simulink library "halin"  (R2021b)
settings: Solver=VariableStepAuto  StartTime=0.0  StopTime=10.0  RelTol=1e-3
undefined symbols (not defined in the file): KHAL_CAN1ABM1E2E_flg, KHAL_CAN1EPB1E2E_flg, KHAL_CAN1EPS1E2E_flg, KHAL_CAN1ESC1E2E_flg, KHAL_CAN1ESC5E2E_flg, KHAL_CAN3BMS1E2E_flg, KHAL_CAN3BMS6E2E_flg, KHAL_CAN3CCU1E2E_flg, KHAL_CAN3CCU2E2E_flg, KHAL_CAN3MCUNF1E2E_flg, KHAL_CAN3MCUNR1E2E_flg, KHAL_CAN3Shifter1E2E_flg, KHAL_CAN3Shifter2E2E_flg, KHAL_CAN6FCM2E2E_flg, KHAL_CAN6FCM4E2E_flg, TRUE
libraries: simulink x645, FVT_lib x212, hcu_lib x59
(part 7 of 23)

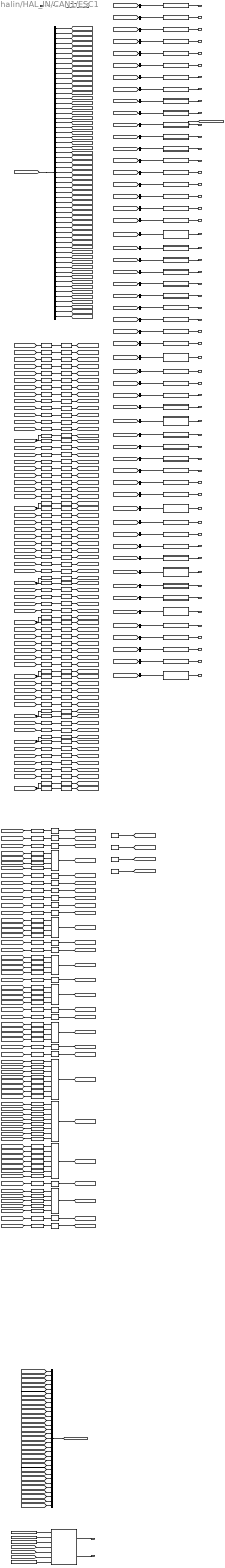
== system halin/HAL_IN/CAN1/ESC1 ==
  DT_CAN1_SG_ESC1 : Inport
  0x5F : Constant  Value=0x5F
  0xB3 : Constant  Value=0xB3
  ABSActive : Subsystem
  ABSFailed : Subsystem
  ABSWnlmpSta : Subsystem
  AVHActive : Subsystem
  AVHFailed : Subsystem
  AmberWnlmpSta : Subsystem
  BTCSActive : Subsystem
  BitwiseAND{,1..66} (67 alike) : simulink/Logic and Bit Operations/Bitwise Operator  logicop=AND  UseBitMask=on  BitMask=0xFF  BitMaskRealWorld=Stored Integer
  BitwiseOR{,1..2,4..9,11..12,14,16..17,19..20,24,26..27} (19 alike) : simulink/Logic and Bit Operations/Bitwise Operator  logicop=OR  UseBitMask=off  BitMask=bin2dec('11011001')  BitMaskRealWorld=Stored Integer
  BitwiseOR{3,10,13,15,18} (5 alike) : simulink/Logic and Bit Operations/Bitwise Operator  logicop=OR  UseBitMask=off  NumInputPorts=4  BitMask=bin2dec('11011001')  BitMaskRealWorld=Stored Integer
  BitwiseOR21 : simulink/Logic and Bit Operations/Bitwise Operator  logicop=OR  UseBitMask=off  NumInputPorts=8  BitMask=bin2dec('11011001')  BitMaskRealWorld=Stored Integer
  BitwiseOR22 : simulink/Logic and Bit Operations/Bitwise Operator  logicop=OR  UseBitMask=off  NumInputPorts=8  BitMask=bin2dec('11011001')  BitMaskRealWorld=Stored Integer
  BitwiseOR23 : simulink/Logic and Bit Operations/Bitwise Operator  logicop=OR  UseBitMask=off  NumInputPorts=7  BitMask=bin2dec('11011001')  BitMaskRealWorld=Stored Integer
  BitwiseOR25 : simulink/Logic and Bit Operations/Bitwise Operator  logicop=OR  UseBitMask=off  NumInputPorts=5  BitMask=bin2dec('11011001')  BitMaskRealWorld=Stored Integer
  DDM_CS&RC_Comparison : FVT_lib/hal/DDM_CS&RC_Comparison  MsgCycleTime=10
  Data Type Conversion{,1..66} (67 alike) : DataTypeConversion  OutDataTypeStr=uint8
  EBDActive : Subsystem
  EBDFailed : Subsystem
  ESC1CS : Subsystem
  ESC1RC : Subsystem
  ESCActive : Subsystem
  ESCBeepReq : Subsystem
  ESCFailed : Subsystem
  ESCOFFStatus : Subsystem
  ESCOfflmpSta : Subsystem
  ESCWnlmpSta : Subsystem
  ESSActive : Subsystem
  FrPTCSActive : Subsystem
  FrntAxlTrqReqDrv : Subsystem
  GRADE : Subsystem
  HBBActive : Subsystem
  HBBFailed : Subsystem
  HDDActive : Subsystem
  HDDFailed : Subsystem
  HSAActive : Subsystem
  HSAFailed : Subsystem
  KHAL_CAN1ESC1E2E_flg : Constant  Value=KHAL_CAN1ESC1E2E_flg
  LFPulseCount : Subsystem
  LFPulseCountV : Subsystem
  LFRawWhlSpeed : Subsystem
  LFRawWhlSpeedV : Subsystem
  LFWhlRotDir : Subsystem
  LRPulseCount : Subsystem
  LRPulseCountV : Subsystem
  LRRawWhlSpeed : Subsystem
  LRRawWhlSpeedV : Subsystem
  LRWhlRotDir : Subsystem
  LeftShift{,6,20,37,40,43} (6 alike) : ArithShift  BitShiftNumber=3  BitShiftDirection=Left
  LeftShift{1,16..17,33..34,36,47} (7 alike) : ArithShift  BitShiftNumber=7  BitShiftDirection=Left
  LeftShift{9..10,18,21,26,28,31..32,38,41..42,45,48,50} (14 alike) : ArithShift  BitShiftDirection=Left
  LeftShift{4,11,24,46} (4 alike) : ArithShift  BitShiftNumber=5  BitShiftDirection=Left
  LeftShift{2,8,12,22,25,44} (6 alike) : ArithShift  BitShiftNumber=6  BitShiftDirection=Left
  LeftShift{13,15,19,27,35,49} (6 alike) : ArithShift  BitShiftNumber=4  BitShiftDirection=Left
  LeftShift14 : ArithShift  BitShiftNumber=1  BitShiftDirection=Left
  LeftShift{5,7,23,29..30,39} (6 alike) : ArithShift  BitShiftNumber=2  BitShiftDirection=Left
  LeftShift3 : ArithShift  BitShiftNumber=1  BitShiftDirection=Left
  MessageRollingCounter : FVT_lib/hal/MessageRollingCounter  CounterMAX=14  task_time_ms=5  msg_time_ms=10
  Mux : Mux  Inputs=31
  PBAActive : Subsystem
  PBAFailed : Subsystem
  RFPulseCount : Subsystem
  RFPulseCountV : Subsystem
  RFRawWhlSpeed : Subsystem
  RFRawWhlSpeedV : Subsystem
  RFWhlRotDir : Subsystem
  RRPulseCount : Subsystem
  RRPulseCountV : Subsystem
  RRRawWhlSpeed : Subsystem
  RRRawWhlSpeedV : Subsystem
  RRWhlRotDir : Subsystem
  RearAxlTrqReqDrv : Subsystem
  RedWnlmpSta : Subsystem
  RightShift{,2,6,10,12} (5 alike) : ArithShift  BitShiftNumber=8
  RightShift{1,3,7,11,13} (5 alike) : ArithShift
  RightShift14 : ArithShift  BitShiftNumber=4
  RightShift15 : ArithShift  BitShiftNumber=-4
  RightShift4 : ArithShift  BitShiftNumber=4
  RightShift5 : ArithShift  BitShiftNumber=-4
  RightShift8 : ArithShift  BitShiftNumber=4
  RightShift9 : ArithShift  BitShiftNumber=-4
  RrPTCSActive : Subsystem
  TCSActive : Subsystem
  TCSFailed : Subsystem
  VehSpeed : Subsystem
  bus_selector : BusSelector  OutputSignals=CAN1_ABS_Active,CAN1_ABS_Failed,CAN1_ABS_WnlmpSta,CAN1_AVH_Active,CAN1_AVH_Failed,CAN1_Amber_WnlmpSta,CAN1_BTCS_Active,CAN1_EBD_Active,CAN1_EBD_Failed,CAN1_ESC1_CS,CAN1_ESC1_RC,CAN1_ESC_Active,CAN1_ESC_BeepReq,CAN1_ESC_EstVehSpd,CAN1_ESC_EstVehSpd_V,CAN1_ESC_Failed,CAN1_ESC_OFF_Status,CAN1_ESC_Off_lmpSta,CAN1_ESC_TSA_Active,CAN1_ESC_WnlmpSta,CAN1_ESS_Active,CAN1_Fr_PTCS_Active,CAN1_FrntAxlTrqReq_Drv,CAN1_GRADE,CAN1_HBB_Active,CAN1_HBB_Failed,CAN1_HDD_Active,CAN1_HDD_Failed,CAN1_HSA_Active,CAN1_HSA_Failed,CAN1_LF_PulseCount,CAN1_LF_PulseCount_V,CAN1_LF_RawWhlSpeed,CAN1_LF_RawWhlSpeed_V,CAN1_LF_WhlRotDir,CAN1_LR_PulseCount,CAN1_LR_PulseCount_V,CAN1_LR_RawWhlSpeed,CAN1_LR_RawWhlSpeed_V,CAN1_LR_WhlRotDir,CAN1_PBA_Active,CAN1_PBA_Failed,CAN1_RF_PulseCount,CAN1_RF_PulseCount_V,CAN1_RF_RawWhlSpeed,CAN1_RF_RawWhlSpeed_V,CAN1_RF_WhlRotDir,CAN1_RR_PulseCount,CAN1_RR_PulseCount_V,CAN1_RR_RawWhlSpeed,CAN1_RR_RawWhlSpeed_V,CAN1_RR_WhlRotDir,CAN1_RearAxlTrqReq_Drv,CAN1_Red_WnlmpSta,CAN1_Rr_PTCS_Active,CAN1_SystemVoltage,CAN1_TCS_Active,CAN1_TCS_Failed,CAN1_VehSpeed
  bus_selector1 : BusSelector  OutputSignals=CAN1_ABS_Active
  bus_selector10 : BusSelector  OutputSignals=CAN1_ESC1_CS
  bus_selector11 : BusSelector  OutputSignals=CAN1_ESC1_RC
  bus_selector12 : BusSelector  OutputSignals=CAN1_ESC_Active
  bus_selector13 : BusSelector  OutputSignals=CAN1_ESC_BeepReq
  bus_selector14 : BusSelector  OutputSignals=CAN1_ESC_Failed
  bus_selector15 : BusSelector  OutputSignals=CAN1_ESC_OFF_Status
  bus_selector16 : BusSelector  OutputSignals=CAN1_ESC_Off_lmpSta
  bus_selector17 : BusSelector  OutputSignals=CAN1_ESC_WnlmpSta
  bus_selector18 : BusSelector  OutputSignals=CAN1_ESS_Active
  bus_selector19 : BusSelector  OutputSignals=CAN1_Fr_PTCS_Active
  bus_selector2 : BusSelector  OutputSignals=CAN1_ABS_Failed
  bus_selector20 : BusSelector  OutputSignals=CAN1_FrntAxlTrqReq_Drv
  bus_selector21 : BusSelector  OutputSignals=CAN1_GRADE
  bus_selector22 : BusSelector  OutputSignals=CAN1_HBB_Active
  bus_selector23 : BusSelector  OutputSignals=CAN1_HBB_Failed
  bus_selector24 : BusSelector  OutputSignals=CAN1_HDD_Active
  bus_selector25 : BusSelector  OutputSignals=CAN1_HDD_Failed
  bus_selector26 : BusSelector  OutputSignals=CAN1_HSA_Active
  bus_selector27 : BusSelector  OutputSignals=CAN1_HSA_Failed
  bus_selector28 : BusSelector  OutputSignals=CAN1_LF_PulseCount
  bus_selector29 : BusSelector  OutputSignals=CAN1_LF_PulseCount_V
  bus_selector3 : BusSelector  OutputSignals=CAN1_ABS_WnlmpSta
  bus_selector30 : BusSelector  OutputSignals=CAN1_LF_RawWhlSpeed
  bus_selector31 : BusSelector  OutputSignals=CAN1_LF_RawWhlSpeed_V
  bus_selector32 : BusSelector  OutputSignals=CAN1_LF_WhlRotDir
  bus_selector33 : BusSelector  OutputSignals=CAN1_LR_PulseCount
  bus_selector34 : BusSelector  OutputSignals=CAN1_LR_PulseCount_V
  bus_selector35 : BusSelector  OutputSignals=CAN1_LR_RawWhlSpeed
  bus_selector36 : BusSelector  OutputSignals=CAN1_LR_RawWhlSpeed_V
  bus_selector37 : BusSelector  OutputSignals=CAN1_LR_WhlRotDir
  bus_selector38 : BusSelector  OutputSignals=CAN1_PBA_Active
  bus_selector39 : BusSelector  OutputSignals=CAN1_PBA_Failed
  bus_selector4 : BusSelector  OutputSignals=CAN1_AVH_Active
  bus_selector40 : BusSelector  OutputSignals=CAN1_RF_PulseCount
  bus_selector41 : BusSelector  OutputSignals=CAN1_RF_PulseCount_V
  bus_selector42 : BusSelector  OutputSignals=CAN1_RF_RawWhlSpeed
  bus_selector43 : BusSelector  OutputSignals=CAN1_RF_RawWhlSpeed_V
  bus_selector44 : BusSelector  OutputSignals=CAN1_RF_WhlRotDir
  bus_selector45 : BusSelector  OutputSignals=CAN1_RR_PulseCount
  bus_selector46 : BusSelector  OutputSignals=CAN1_RR_PulseCount_V
  bus_selector47 : BusSelector  OutputSignals=CAN1_RR_RawWhlSpeed
  bus_selector48 : BusSelector  OutputSignals=CAN1_RR_RawWhlSpeed_V
  bus_selector49 : BusSelector  OutputSignals=CAN1_RR_WhlRotDir
  bus_selector5 : BusSelector  OutputSignals=CAN1_AVH_Failed
  bus_selector50 : BusSelector  OutputSignals=CAN1_RearAxlTrqReq_Drv
  bus_selector51 : BusSelector  OutputSignals=CAN1_Red_WnlmpSta
  bus_selector52 : BusSelector  OutputSignals=CAN1_Rr_PTCS_Active
  bus_selector53 : BusSelector  OutputSignals=CAN1_TCS_Active
  bus_selector54 : BusSelector  OutputSignals=CAN1_TCS_Failed
  bus_selector55 : BusSelector  OutputSignals=CAN1_VehSpeed
  bus_selector6 : BusSelector  OutputSignals=CAN1_Amber_WnlmpSta
  bus_selector7 : BusSelector  OutputSignals=CAN1_BTCS_Active
  bus_selector8 : BusSelector  OutputSignals=CAN1_EBD_Active
  bus_selector9 : BusSelector  OutputSignals=CAN1_EBD_Failed
  constant{,1..3} (4 alike) : Constant  Value=0x0  OutDataTypeStr=uint8
  VHAL_ESC1CSErr_flg : Outport
  VHAL_ESC1RCErr_flg : Outport  Port=2
  VHAL_ABSActive_flg : Outport  Port=3
  VHAL_ABSFailed_flg : Outport  Port=4
  VHAL_ABSWnlmpSta_flg : Outport  Port=5
  VHAL_AVHActive_flg : Outport  Port=6
  VHAL_AVHFailed_flg : Outport  Port=7
  VHAL_AmberWnlmpSta_flg : Outport  Port=8
  VHAL_BTCSActive_flg : Outport  Port=9
  VHAL_EBDActive_flg : Outport  Port=10
  VHAL_EBDFailed_flg : Outport  Port=11
  VHAL_ESC1CS_enum : Outport  Port=12
  VHAL_ESC1RC_enum : Outport  Port=13
  VHAL_ESCActive_flg : Outport  Port=14
  VHAL_ESCBeepReq_flg : Outport  Port=15
  VHAL_ESCFailed_flg : Outport  Port=16
  VHAL_ESCOFFStatus_enum : Outport  Port=17
  VHAL_ESCOfflmpSta_flg : Outport  Port=18
  VHAL_ESCWnlmpSta_enum : Outport  Port=19
  VHAL_ESSActive_flg : Outport  Port=20
  VHAL_FrPTCSActive_flg : Outport  Port=21
  VHAL_FrntAxlTrqReqDrv_Nm : Outport  Port=22
  VHAL_GRADE_Deg : Outport  Port=23
  VHAL_HBBActive_flg : Outport  Port=24
  VHAL_HBBFailed_flg : Outport  Port=25
  VHAL_HDDActive_flg : Outport  Port=26
  VHAL_HDDFailed_flg : Outport  Port=27
  VHAL_HSAActive_flg : Outport  Port=28
  VHAL_HSAFailed_flg : Outport  Port=29
  VHAL_LFPulseCount_enum : Outport  Port=30
  VHAL_LFPulseCountV_flg : Outport  Port=31
  VHAL_LFRawWhlSpeed_kph : Outport  Port=32
  VHAL_LFRawWhlSpeedV_flg : Outport  Port=33
  VHAL_LFWhlRotDir_enum : Outport  Port=34
  VHAL_LRPulseCount_enum : Outport  Port=35
  VHAL_LRPulseCountV_flg : Outport  Port=36
  VHAL_LRRawWhlSpeed_kph : Outport  Port=37
  VHAL_LRRawWhlSpeedV_flg : Outport  Port=38
  VHAL_LRWhlRotDir_enum : Outport  Port=39
  VHAL_PBAActive_flg : Outport  Port=40
  VHAL_PBAFailed_flg : Outport  Port=41
  VHAL_RFPulseCount_enum : Outport  Port=42
  VHAL_RFPulseCountV_flg : Outport  Port=43
  VHAL_RFRawWhlSpeed_kph : Outport  Port=44
  VHAL_RFRawWhlSpeedV_flg : Outport  Port=45
  VHAL_RFWhlRotDir_enum : Outport  Port=46
  VHAL_RRPulseCount_enum : Outport  Port=47
  VHAL_RRPulseCountV_flg : Outport  Port=48
  VHAL_RRRawWhlSpeed_kph : Outport  Port=49
  VHAL_RRRawWhlSpeedV_flg : Outport  Port=50
  VHAL_RRWhlRotDir_enum : Outport  Port=51
  VHAL_RearAxlTrqReqDrv_Nm : Outport  Port=52
  VHAL_RedWnlmpSta_flg : Outport  Port=53
  VHAL_RrPTCSActive_flg : Outport  Port=54
  VHAL_TCSActive_flg : Outport  Port=55
  VHAL_TCSFailed_flg : Outport  Port=56
  VHAL_VehSpeed_kph : Outport  Port=57
  wires:
  DT_CAN1_SG_ESC1/1 -> [DT_CAN1_SG_ESC1]
  [DT_CAN1_SG_ESC1] -> bus_selector/1
  bus_selector/1 -> [CAN1_ABS_Active]  "<CAN1_ABS_Active>"
  [CAN1_ABS_Active] -> LeftShift/1
  LeftShift/1 -> BitwiseAND/1
  BitwiseAND/1 -> [Byte_23_CAN1_ABS_Active]
  bus_selector/2 -> [CAN1_ABS_Failed]  "<CAN1_ABS_Failed>"
  [CAN1_ABS_Failed] -> LeftShift1/1
  LeftShift1/1 -> BitwiseAND1/1
  BitwiseAND1/1 -> [Byte_22_CAN1_ABS_Failed]
  bus_selector/3 -> [CAN1_ABS_WnlmpSta]  "<CAN1_ABS_WnlmpSta>"
  [CAN1_ABS_WnlmpSta] -> LeftShift2/1
  LeftShift2/1 -> BitwiseAND2/1
  BitwiseAND2/1 -> [Byte_25_CAN1_ABS_WnlmpSta]
  bus_selector/4 -> [CAN1_AVH_Active]  "<CAN1_AVH_Active>"
  [CAN1_AVH_Active] -> LeftShift3/1
  LeftShift3/1 -> BitwiseAND3/1
  BitwiseAND3/1 -> [Byte_22_CAN1_AVH_Active]
  bus_selector/5 -> [CAN1_AVH_Failed]  "<CAN1_AVH_Failed>"
  [CAN1_AVH_Failed] -> LeftShift4/1
  LeftShift4/1 -> BitwiseAND4/1
  BitwiseAND4/1 -> [Byte_21_CAN1_AVH_Failed]
  bus_selector/6 -> [CAN1_Amber_WnlmpSta]  "<CAN1_Amber_WnlmpSta>"
  [CAN1_Amber_WnlmpSta] -> LeftShift5/1
  LeftShift5/1 -> BitwiseAND5/1
  BitwiseAND5/1 -> [Byte_22_CAN1_Amber_WnlmpSta]
  bus_selector/7 -> [CAN1_BTCS_Active]  "<CAN1_BTCS_Active>"
  [CAN1_BTCS_Active] -> LeftShift6/1
  LeftShift6/1 -> BitwiseAND6/1
  BitwiseAND6/1 -> [Byte_22_CAN1_BTCS_Active]
  bus_selector/8 -> [CAN1_EBD_Active]  "<CAN1_EBD_Active>"
  [CAN1_EBD_Active] -> LeftShift7/1
  LeftShift7/1 -> BitwiseAND7/1
  BitwiseAND7/1 -> [Byte_23_CAN1_EBD_Active]
  bus_selector/9 -> [CAN1_EBD_Failed]  "<CAN1_EBD_Failed>"
  [CAN1_EBD_Failed] -> LeftShift8/1
  LeftShift8/1 -> BitwiseAND8/1
  BitwiseAND8/1 -> [Byte_22_CAN1_EBD_Failed]
  bus_selector/10 -> [CAN1_ESC1_CS]  "<CAN1_ESC1_CS>"
  [CAN1_ESC1_CS] -> LeftShift9/1
  LeftShift9/1 -> BitwiseAND9/1
  BitwiseAND9/1 -> [Byte_0_CAN1_ESC1_CS]
  bus_selector/11 -> [CAN1_ESC1_RC]  "<CAN1_ESC1_RC>"
  [CAN1_ESC1_RC] -> LeftShift10/1
  LeftShift10/1 -> BitwiseAND10/1
  BitwiseAND10/1 -> [Byte_1_CAN1_ESC1_RC]
  bus_selector/12 -> [CAN1_ESC_Active]  "<CAN1_ESC_Active>"
  [CAN1_ESC_Active] -> LeftShift11/1
  LeftShift11/1 -> BitwiseAND11/1
  BitwiseAND11/1 -> [Byte_23_CAN1_ESC_Active]
  bus_selector/13 -> [CAN1_ESC_BeepReq]  "<CAN1_ESC_BeepReq>"
  [CAN1_ESC_BeepReq] -> LeftShift12/1
  LeftShift12/1 -> BitwiseAND12/1
  BitwiseAND12/1 -> [Byte_18_CAN1_ESC_BeepReq]
  bus_selector/14 -> [CAN1_ESC_EstVehSpd]  "<CAN1_ESC_EstVehSpd>"
  [CAN1_ESC_EstVehSpd] -> RightShift/1, RightShift1/1
  RightShift/1 -> BitwiseAND13/1
  BitwiseAND13/1 -> [Byte_25_CAN1_ESC_EstVehSpd]
  RightShift1/1 -> BitwiseAND14/1
  BitwiseAND14/1 -> [Byte_26_CAN1_ESC_EstVehSpd]
  bus_selector/15 -> [CAN1_ESC_EstVehSpd_V]  "<CAN1_ESC_EstVehSpd_V>"
  [CAN1_ESC_EstVehSpd_V] -> LeftShift13/1
  LeftShift13/1 -> BitwiseAND15/1
  BitwiseAND15/1 -> [Byte_25_CAN1_ESC_EstVehSpd_V]
  bus_selector/16 -> [CAN1_ESC_Failed]  "<CAN1_ESC_Failed>"
  [CAN1_ESC_Failed] -> LeftShift14/1
  LeftShift14/1 -> BitwiseAND16/1
  BitwiseAND16/1 -> [Byte_21_CAN1_ESC_Failed]
  bus_selector/17 -> [CAN1_ESC_OFF_Status]  "<CAN1_ESC_OFF_Status>"
  [CAN1_ESC_OFF_Status] -> LeftShift15/1
  LeftShift15/1 -> BitwiseAND17/1
  BitwiseAND17/1 -> [Byte_18_CAN1_ESC_OFF_Status]
  bus_selector/18 -> [CAN1_ESC_Off_lmpSta]  "<CAN1_ESC_Off_lmpSta>"
  [CAN1_ESC_Off_lmpSta] -> LeftShift16/1
  LeftShift16/1 -> BitwiseAND18/1
  BitwiseAND18/1 -> [Byte_25_CAN1_ESC_Off_lmpSta]
  bus_selector/19 -> [CAN1_ESC_TSA_Active]  "<CAN1_ESC_TSA_Active>"
  [CAN1_ESC_TSA_Active] -> LeftShift17/1
  LeftShift17/1 -> BitwiseAND19/1
  BitwiseAND19/1 -> [Byte_27_CAN1_ESC_TSA_Active]
  bus_selector/20 -> [CAN1_ESC_WnlmpSta]  "<CAN1_ESC_WnlmpSta>"
  [CAN1_ESC_WnlmpSta] -> LeftShift18/1
  LeftShift18/1 -> BitwiseAND20/1
  BitwiseAND20/1 -> [Byte_23_CAN1_ESC_WnlmpSta]
  bus_selector/21 -> [CAN1_ESS_Active]  "<CAN1_ESS_Active>"
  [CAN1_ESS_Active] -> LeftShift19/1
  LeftShift19/1 -> BitwiseAND21/1
  BitwiseAND21/1 -> [Byte_22_CAN1_ESS_Active]
  bus_selector/22 -> [CAN1_Fr_PTCS_Active]  "<CAN1_Fr_PTCS_Active>"
  [CAN1_Fr_PTCS_Active] -> LeftShift20/1
  LeftShift20/1 -> BitwiseAND22/1
  BitwiseAND22/1 -> [Byte_3_CAN1_Fr_PTCS_Active]
  bus_selector/23 -> [CAN1_FrntAxlTrqReq_Drv]  "<CAN1_FrntAxlTrqReq_Drv>"
  [CAN1_FrntAxlTrqReq_Drv] -> RightShift2/1, RightShift3/1
  RightShift2/1 -> BitwiseAND23/1
  BitwiseAND23/1 -> [Byte_4_CAN1_FrntAxlTrqReq_Drv]
  RightShift3/1 -> BitwiseAND24/1
  BitwiseAND24/1 -> [Byte_5_CAN1_FrntAxlTrqReq_Drv]
  bus_selector/24 -> [CAN1_GRADE]  "<CAN1_GRADE>"
  [CAN1_GRADE] -> LeftShift21/1
  LeftShift21/1 -> BitwiseAND25/1
  BitwiseAND25/1 -> [Byte_24_CAN1_GRADE]
  bus_selector/25 -> [CAN1_HBB_Active]  "<CAN1_HBB_Active>"
  [CAN1_HBB_Active] -> LeftShift22/1
  LeftShift22/1 -> BitwiseAND26/1
  BitwiseAND26/1 -> [Byte_23_CAN1_HBB_Active]
  bus_selector/26 -> [CAN1_HBB_Failed]  "<CAN1_HBB_Failed>"
  [CAN1_HBB_Failed] -> LeftShift23/1
  LeftShift23/1 -> BitwiseAND27/1
  BitwiseAND27/1 -> [Byte_21_CAN1_HBB_Failed]
  bus_selector/27 -> [CAN1_HDD_Active]  "<CAN1_HDD_Active>"
  [CAN1_HDD_Active] -> LeftShift24/1
  LeftShift24/1 -> BitwiseAND28/1
  BitwiseAND28/1 -> [Byte_22_CAN1_HDD_Active]
  bus_selector/28 -> [CAN1_HDD_Failed]  "<CAN1_HDD_Failed>"
  [CAN1_HDD_Failed] -> LeftShift25/1
  LeftShift25/1 -> BitwiseAND29/1
  BitwiseAND29/1 -> [Byte_21_CAN1_HDD_Failed]
  bus_selector/29 -> [CAN1_HSA_Active]  "<CAN1_HSA_Active>"
  [CAN1_HSA_Active] -> LeftShift26/1
  LeftShift26/1 -> BitwiseAND30/1
  BitwiseAND30/1 -> [Byte_22_CAN1_HSA_Active]
  bus_selector/30 -> [CAN1_HSA_Failed]  "<CAN1_HSA_Failed>"
  [CAN1_HSA_Failed] -> LeftShift27/1
  LeftShift27/1 -> BitwiseAND31/1
  BitwiseAND31/1 -> [Byte_21_CAN1_HSA_Failed]
  bus_selector/31 -> [CAN1_LF_PulseCount]  "<CAN1_LF_PulseCount>"
  [CAN1_LF_PulseCount] -> LeftShift28/1
  LeftShift28/1 -> BitwiseAND32/1
  BitwiseAND32/1 -> [Byte_11_CAN1_LF_PulseCount]
  bus_selector/32 -> [CAN1_LF_PulseCount_V]  "<CAN1_LF_PulseCount_V>"
  [CAN1_LF_PulseCount_V] -> LeftShift29/1
  LeftShift29/1 -> BitwiseAND33/1
  BitwiseAND33/1 -> [Byte_10_CAN1_LF_PulseCount_V]
  bus_selector/33 -> [CAN1_LF_RawWhlSpeed]  "<CAN1_LF_RawWhlSpeed>"
  [CAN1_LF_RawWhlSpeed] -> RightShift4/1, RightShift5/1
  RightShift4/1 -> BitwiseAND34/1
  BitwiseAND34/1 -> [Byte_12_CAN1_LF_RawWhlSpeed]
  RightShift5/1 -> BitwiseAND35/1
  BitwiseAND35/1 -> [Byte_13_CAN1_LF_RawWhlSpeed]
  bus_selector/34 -> [CAN1_LF_RawWhlSpeed_V]  "<CAN1_LF_RawWhlSpeed_V>"
  [CAN1_LF_RawWhlSpeed_V] -> LeftShift30/1
  LeftShift30/1 -> BitwiseAND36/1
  BitwiseAND36/1 -> [Byte_13_CAN1_LF_RawWhlSpeed_V]
  bus_selector/35 -> [CAN1_LF_WhlRotDir]  "<CAN1_LF_WhlRotDir>"
  [CAN1_LF_WhlRotDir] -> LeftShift31/1
  LeftShift31/1 -> BitwiseAND37/1
  BitwiseAND37/1 -> [Byte_10_CAN1_LF_WhlRotDir]
  bus_selector/36 -> [CAN1_LR_PulseCount]  "<CAN1_LR_PulseCount>"
  [CAN1_LR_PulseCount] -> LeftShift32/1
  LeftShift32/1 -> BitwiseAND38/1
  BitwiseAND38/1 -> [Byte_17_CAN1_LR_PulseCount]
  bus_selector/37 -> [CAN1_LR_PulseCount_V]  "<CAN1_LR_PulseCount_V>"
  [CAN1_LR_PulseCount_V] -> LeftShift33/1
  LeftShift33/1 -> BitwiseAND39/1
  BitwiseAND39/1 -> [Byte_15_CAN1_LR_PulseCount_V]
  bus_selector/38 -> [CAN1_LR_RawWhlSpeed]  "<CAN1_LR_RawWhlSpeed>"
  [CAN1_LR_RawWhlSpeed] -> RightShift6/1, RightShift7/1
  RightShift6/1 -> BitwiseAND40/1
  BitwiseAND40/1 -> [Byte_18_CAN1_LR_RawWhlSpeed]
  RightShift7/1 -> BitwiseAND41/1
  BitwiseAND41/1 -> [Byte_19_CAN1_LR_RawWhlSpeed]
  bus_selector/39 -> [CAN1_LR_RawWhlSpeed_V]  "<CAN1_LR_RawWhlSpeed_V>"
  [CAN1_LR_RawWhlSpeed_V] -> LeftShift34/1
  LeftShift34/1 -> BitwiseAND42/1
  BitwiseAND42/1 -> [Byte_18_CAN1_LR_RawWhlSpeed_V]
  bus_selector/40 -> [CAN1_LR_WhlRotDir]  "<CAN1_LR_WhlRotDir>"
  [CAN1_LR_WhlRotDir] -> LeftShift35/1
  LeftShift35/1 -> BitwiseAND43/1
  BitwiseAND43/1 -> [Byte_15_CAN1_LR_WhlRotDir]
  bus_selector/41 -> [CAN1_PBA_Active]  "<CAN1_PBA_Active>"
  [CAN1_PBA_Active] -> LeftShift36/1
  LeftShift36/1 -> BitwiseAND44/1
  BitwiseAND44/1 -> [Byte_23_CAN1_PBA_Active]
  bus_selector/42 -> [CAN1_PBA_Failed]  "<CAN1_PBA_Failed>"
  [CAN1_PBA_Failed] -> LeftShift37/1
  LeftShift37/1 -> BitwiseAND45/1
  BitwiseAND45/1 -> [Byte_21_CAN1_PBA_Failed]
  bus_selector/43 -> [CAN1_RF_PulseCount]  "<CAN1_RF_PulseCount>"
  [CAN1_RF_PulseCount] -> LeftShift38/1
  LeftShift38/1 -> BitwiseAND46/1
  BitwiseAND46/1 -> [Byte_8_CAN1_RF_PulseCount]
  bus_selector/44 -> [CAN1_RF_PulseCount_V]  "<CAN1_RF_PulseCount_V>"
  [CAN1_RF_PulseCount_V] -> LeftShift39/1
  LeftShift39/1 -> BitwiseAND47/1
  BitwiseAND47/1 -> [Byte_3_CAN1_RF_PulseCount_V]
  bus_selector/45 -> [CAN1_RF_RawWhlSpeed]  "<CAN1_RF_RawWhlSpeed>"
  [CAN1_RF_RawWhlSpeed] -> RightShift8/1, RightShift9/1
  RightShift8/1 -> BitwiseAND48/1
  BitwiseAND48/1 -> [Byte_9_CAN1_RF_RawWhlSpeed]
  RightShift9/1 -> BitwiseAND49/1
  BitwiseAND49/1 -> [Byte_10_CAN1_RF_RawWhlSpeed]
  bus_selector/46 -> [CAN1_RF_RawWhlSpeed_V]  "<CAN1_RF_RawWhlSpeed_V>"
  [CAN1_RF_RawWhlSpeed_V] -> LeftShift40/1
  LeftShift40/1 -> BitwiseAND50/1
  BitwiseAND50/1 -> [Byte_10_CAN1_RF_RawWhlSpeed_V]
  bus_selector/47 -> [CAN1_RF_WhlRotDir]  "<CAN1_RF_WhlRotDir>"
  [CAN1_RF_WhlRotDir] -> LeftShift41/1
  LeftShift41/1 -> BitwiseAND51/1
  BitwiseAND51/1 -> [Byte_3_CAN1_RF_WhlRotDir]
  bus_selector/48 -> [CAN1_RR_PulseCount]  "<CAN1_RR_PulseCount>"
  [CAN1_RR_PulseCount] -> LeftShift42/1
  LeftShift42/1 -> BitwiseAND52/1
  BitwiseAND52/1 -> [Byte_14_CAN1_RR_PulseCount]
  bus_selector/49 -> [CAN1_RR_PulseCount_V]  "<CAN1_RR_PulseCount_V>"
  [CAN1_RR_PulseCount_V] -> LeftShift43/1
  LeftShift43/1 -> BitwiseAND53/1
  BitwiseAND53/1 -> [Byte_13_CAN1_RR_PulseCount_V]
  bus_selector/50 -> [CAN1_RR_RawWhlSpeed]  "<CAN1_RR_RawWhlSpeed>"
  [CAN1_RR_RawWhlSpeed] -> RightShift10/1, RightShift11/1
  RightShift10/1 -> BitwiseAND54/1
  BitwiseAND54/1 -> [Byte_15_CAN1_RR_RawWhlSpeed]
  RightShift11/1 -> BitwiseAND55/1
  BitwiseAND55/1 -> [Byte_16_CAN1_RR_RawWhlSpeed]
  bus_selector/51 -> [CAN1_RR_RawWhlSpeed_V]  "<CAN1_RR_RawWhlSpeed_V>"
  [CAN1_RR_RawWhlSpeed_V] -> LeftShift44/1
  LeftShift44/1 -> BitwiseAND56/1
  BitwiseAND56/1 -> [Byte_15_CAN1_RR_RawWhlSpeed_V]
  bus_selector/52 -> [CAN1_RR_WhlRotDir]  "<CAN1_RR_WhlRotDir>"
  [CAN1_RR_WhlRotDir] -> LeftShift45/1
  LeftShift45/1 -> BitwiseAND57/1
  BitwiseAND57/1 -> [Byte_13_CAN1_RR_WhlRotDir]
  bus_selector/53 -> [CAN1_RearAxlTrqReq_Drv]  "<CAN1_RearAxlTrqReq_Drv>"
  [CAN1_RearAxlTrqReq_Drv] -> RightShift12/1, RightShift13/1
  RightShift12/1 -> BitwiseAND58/1
  BitwiseAND58/1 -> [Byte_6_CAN1_RearAxlTrqReq_Drv]
  RightShift13/1 -> BitwiseAND59/1
  BitwiseAND59/1 -> [Byte_7_CAN1_RearAxlTrqReq_Drv]
  bus_selector/54 -> [CAN1_Red_WnlmpSta]  "<CAN1_Red_WnlmpSta>"
  [CAN1_Red_WnlmpSta] -> LeftShift46/1
  LeftShift46/1 -> BitwiseAND60/1
  BitwiseAND60/1 -> [Byte_25_CAN1_Red_WnlmpSta]
  bus_selector/55 -> [CAN1_Rr_PTCS_Active]  "<CAN1_Rr_PTCS_Active>"
  [CAN1_Rr_PTCS_Active] -> LeftShift47/1
  LeftShift47/1 -> BitwiseAND61/1
  BitwiseAND61/1 -> [Byte_21_CAN1_Rr_PTCS_Active]
  bus_selector/56 -> [CAN1_SystemVoltage]  "<CAN1_SystemVoltage>"
  [CAN1_SystemVoltage] -> LeftShift48/1
  LeftShift48/1 -> BitwiseAND62/1
  BitwiseAND62/1 -> [Byte_20_CAN1_SystemVoltage]
  bus_selector/57 -> [CAN1_TCS_Active]  "<CAN1_TCS_Active>"
  [CAN1_TCS_Active] -> LeftShift49/1
  LeftShift49/1 -> BitwiseAND63/1
  BitwiseAND63/1 -> [Byte_23_CAN1_TCS_Active]
  bus_selector/58 -> [CAN1_TCS_Failed]  "<CAN1_TCS_Failed>"
  [CAN1_TCS_Failed] -> LeftShift50/1
  LeftShift50/1 -> BitwiseAND64/1
  BitwiseAND64/1 -> [Byte_21_CAN1_TCS_Failed]
  bus_selector/59 -> [CAN1_VehSpeed]  "<CAN1_VehSpeed>"
  [CAN1_VehSpeed] -> RightShift14/1, RightShift15/1
  RightShift14/1 -> BitwiseAND65/1
  BitwiseAND65/1 -> [Byte_2_CAN1_VehSpeed]
  RightShift15/1 -> BitwiseAND66/1
  BitwiseAND66/1 -> [Byte_3_CAN1_VehSpeed]
  Data Type Conversion/1 -> BitwiseOR/1
  [Byte_0_CAN1_ESC1_CS] -> Data Type Conversion/1
  BitwiseOR/1 -> [Byte_0]
  Data Type Conversion1/1 -> BitwiseOR1/1
  [Byte_1_CAN1_ESC1_RC] -> Data Type Conversion1/1
  BitwiseOR1/1 -> [Byte_1]
  Data Type Conversion2/1 -> BitwiseOR2/1
  [Byte_2_CAN1_VehSpeed] -> Data Type Conversion2/1
  BitwiseOR2/1 -> [Byte_2]
  Data Type Conversion3/1 -> BitwiseOR3/1
  [Byte_3_CAN1_Fr_PTCS_Active] -> Data Type Conversion3/1
  Data Type Conversion4/1 -> BitwiseOR3/2
  [Byte_3_CAN1_RF_PulseCount_V] -> Data Type Conversion4/1
  Data Type Conversion5/1 -> BitwiseOR3/3
  [Byte_3_CAN1_RF_WhlRotDir] -> Data Type Conversion5/1
  Data Type Conversion6/1 -> BitwiseOR3/4
  [Byte_3_CAN1_VehSpeed] -> Data Type Conversion6/1
  BitwiseOR3/1 -> [Byte_3]
  Data Type Conversion7/1 -> BitwiseOR4/1
  [Byte_4_CAN1_FrntAxlTrqReq_Drv] -> Data Type Conversion7/1
  BitwiseOR4/1 -> [Byte_4]
  Data Type Conversion8/1 -> BitwiseOR5/1
  [Byte_5_CAN1_FrntAxlTrqReq_Drv] -> Data Type Conversion8/1
  BitwiseOR5/1 -> [Byte_5]
  Data Type Conversion9/1 -> BitwiseOR6/1
  [Byte_6_CAN1_RearAxlTrqReq_Drv] -> Data Type Conversion9/1
  BitwiseOR6/1 -> [Byte_6]
  Data Type Conversion10/1 -> BitwiseOR7/1
  [Byte_7_CAN1_RearAxlTrqReq_Drv] -> Data Type Conversion10/1
  BitwiseOR7/1 -> [Byte_7]
  Data Type Conversion11/1 -> BitwiseOR8/1
  [Byte_8_CAN1_RF_PulseCount] -> Data Type Conversion11/1
  BitwiseOR8/1 -> [Byte_8]
  Data Type Conversion12/1 -> BitwiseOR9/1
  [Byte_9_CAN1_RF_RawWhlSpeed] -> Data Type Conversion12/1
  BitwiseOR9/1 -> [Byte_9]
  Data Type Conversion13/1 -> BitwiseOR10/1
  [Byte_10_CAN1_LF_PulseCount_V] -> Data Type Conversion13/1
  Data Type Conversion14/1 -> BitwiseOR10/2
  [Byte_10_CAN1_LF_WhlRotDir] -> Data Type Conversion14/1
  Data Type Conversion15/1 -> BitwiseOR10/3
  [Byte_10_CAN1_RF_RawWhlSpeed] -> Data Type Conversion15/1
  Data Type Conversion16/1 -> BitwiseOR10/4
  [Byte_10_CAN1_RF_RawWhlSpeed_V] -> Data Type Conversion16/1
  BitwiseOR10/1 -> [Byte_10]
  Data Type Conversion17/1 -> BitwiseOR11/1
  [Byte_11_CAN1_LF_PulseCount] -> Data Type Conversion17/1
  BitwiseOR11/1 -> [Byte_11]
  Data Type Conversion18/1 -> BitwiseOR12/1
  [Byte_12_CAN1_LF_RawWhlSpeed] -> Data Type Conversion18/1
  BitwiseOR12/1 -> [Byte_12]
  Data Type Conversion19/1 -> BitwiseOR13/1
  [Byte_13_CAN1_LF_RawWhlSpeed] -> Data Type Conversion19/1
  Data Type Conversion20/1 -> BitwiseOR13/2
  [Byte_13_CAN1_LF_RawWhlSpeed_V] -> Data Type Conversion20/1
  Data Type Conversion21/1 -> BitwiseOR13/3
  [Byte_13_CAN1_RR_PulseCount_V] -> Data Type Conversion21/1
  Data Type Conversion22/1 -> BitwiseOR13/4
  [Byte_13_CAN1_RR_WhlRotDir] -> Data Type Conversion22/1
  BitwiseOR13/1 -> [Byte_13]
  Data Type Conversion23/1 -> BitwiseOR14/1
  [Byte_14_CAN1_RR_PulseCount] -> Data Type Conversion23/1
  BitwiseOR14/1 -> [Byte_14]
  Data Type Conversion24/1 -> BitwiseOR15/1
  [Byte_15_CAN1_LR_PulseCount_V] -> Data Type Conversion24/1
  Data Type Conversion25/1 -> BitwiseOR15/2
  [Byte_15_CAN1_LR_WhlRotDir] -> Data Type Conversion25/1
  Data Type Conversion26/1 -> BitwiseOR15/3
  [Byte_15_CAN1_RR_RawWhlSpeed] -> Data Type Conversion26/1
  Data Type Conversion27/1 -> BitwiseOR15/4
  [Byte_15_CAN1_RR_RawWhlSpeed_V] -> Data Type Conversion27/1
  BitwiseOR15/1 -> [Byte_15]
  Data Type Conversion28/1 -> BitwiseOR16/1
  [Byte_16_CAN1_RR_RawWhlSpeed] -> Data Type Conversion28/1
  BitwiseOR16/1 -> [Byte_16]
  Data Type Conversion29/1 -> BitwiseOR17/1
  [Byte_17_CAN1_LR_PulseCount] -> Data Type Conversion29/1
  BitwiseOR17/1 -> [Byte_17]
  Data Type Conversion30/1 -> BitwiseOR18/1
  [Byte_18_CAN1_ESC_BeepReq] -> Data Type Conversion30/1
  Data Type Conversion31/1 -> BitwiseOR18/2
  [Byte_18_CAN1_ESC_OFF_Status] -> Data Type Conversion31/1
  Data Type Conversion32/1 -> BitwiseOR18/3
  [Byte_18_CAN1_LR_RawWhlSpeed] -> Data Type Conversion32/1
  Data Type Conversion33/1 -> BitwiseOR18/4
  [Byte_18_CAN1_LR_RawWhlSpeed_V] -> Data Type Conversion33/1
  BitwiseOR18/1 -> [Byte_18]
  Data Type Conversion34/1 -> BitwiseOR19/1
  [Byte_19_CAN1_LR_RawWhlSpeed] -> Data Type Conversion34/1
  BitwiseOR19/1 -> [Byte_19]
  Data Type Conversion35/1 -> BitwiseOR20/1
  [Byte_20_CAN1_SystemVoltage] -> Data Type Conversion35/1
  BitwiseOR20/1 -> [Byte_20]
  Data Type Conversion36/1 -> BitwiseOR21/1
  [Byte_21_CAN1_AVH_Failed] -> Data Type Conversion36/1
  Data Type Conversion37/1 -> BitwiseOR21/2
  [Byte_21_CAN1_ESC_Failed] -> Data Type Conversion37/1
  Data Type Conversion38/1 -> BitwiseOR21/3
  [Byte_21_CAN1_HBB_Failed] -> Data Type Conversion38/1
  Data Type Conversion39/1 -> BitwiseOR21/4
  [Byte_21_CAN1_HDD_Failed] -> Data Type Conversion39/1
  Data Type Conversion40/1 -> BitwiseOR21/5
  [Byte_21_CAN1_HSA_Failed] -> Data Type Conversion40/1
  Data Type Conversion41/1 -> BitwiseOR21/6
  [Byte_21_CAN1_PBA_Failed] -> Data Type Conversion41/1
  Data Type Conversion42/1 -> BitwiseOR21/7
  [Byte_21_CAN1_Rr_PTCS_Active] -> Data Type Conversion42/1
  Data Type Conversion43/1 -> BitwiseOR21/8
  [Byte_21_CAN1_TCS_Failed] -> Data Type Conversion43/1
  BitwiseOR21/1 -> [Byte_21]
  Data Type Conversion44/1 -> BitwiseOR22/1
  [Byte_22_CAN1_ABS_Failed] -> Data Type Conversion44/1
  Data Type Conversion45/1 -> BitwiseOR22/2
  [Byte_22_CAN1_AVH_Active] -> Data Type Conversion45/1
  Data Type Conversion46/1 -> BitwiseOR22/3
  [Byte_22_CAN1_Amber_WnlmpSta] -> Data Type Conversion46/1
  Data Type Conversion47/1 -> BitwiseOR22/4
  [Byte_22_CAN1_BTCS_Active] -> Data Type Conversion47/1
  Data Type Conversion48/1 -> BitwiseOR22/5
  [Byte_22_CAN1_EBD_Failed] -> Data Type Conversion48/1
  Data Type Conversion49/1 -> BitwiseOR22/6
  [Byte_22_CAN1_ESS_Active] -> Data Type Conversion49/1
  Data Type Conversion50/1 -> BitwiseOR22/7
  [Byte_22_CAN1_HDD_Active] -> Data Type Conversion50/1
  Data Type Conversion51/1 -> BitwiseOR22/8
  [Byte_22_CAN1_HSA_Active] -> Data Type Conversion51/1
  BitwiseOR22/1 -> [Byte_22]
  Data Type Conversion52/1 -> BitwiseOR23/1
  [Byte_23_CAN1_ABS_Active] -> Data Type Conversion52/1
  Data Type Conversion53/1 -> BitwiseOR23/2
  [Byte_23_CAN1_EBD_Active] -> Data Type Conversion53/1
  Data Type Conversion54/1 -> BitwiseOR23/3
  [Byte_23_CAN1_ESC_Active] -> Data Type Conversion54/1
  Data Type Conversion55/1 -> BitwiseOR23/4
  [Byte_23_CAN1_ESC_WnlmpSta] -> Data Type Conversion55/1
  Data Type Conversion56/1 -> BitwiseOR23/5
  [Byte_23_CAN1_HBB_Active] -> Data Type Conversion56/1
  Data Type Conversion57/1 -> BitwiseOR23/6
  [Byte_23_CAN1_PBA_Active] -> Data Type Conversion57/1
  Data Type Conversion58/1 -> BitwiseOR23/7
  [Byte_23_CAN1_TCS_Active] -> Data Type Conversion58/1
  BitwiseOR23/1 -> [Byte_23]
  Data Type Conversion59/1 -> BitwiseOR24/1
  [Byte_24_CAN1_GRADE] -> Data Type Conversion59/1
  BitwiseOR24/1 -> [Byte_24]
  Data Type Conversion60/1 -> BitwiseOR25/1
  [Byte_25_CAN1_ABS_WnlmpSta] -> Data Type Conversion60/1
  Data Type Conversion61/1 -> BitwiseOR25/2
  [Byte_25_CAN1_ESC_EstVehSpd] -> Data Type Conversion61/1
  Data Type Conversion62/1 -> BitwiseOR25/3
  [Byte_25_CAN1_ESC_EstVehSpd_V] -> Data Type Conversion62/1
  Data Type Conversion63/1 -> BitwiseOR25/4
  [Byte_25_CAN1_ESC_Off_lmpSta] -> Data Type Conversion63/1
  Data Type Conversion64/1 -> BitwiseOR25/5
  [Byte_25_CAN1_Red_WnlmpSta] -> Data Type Conversion64/1
  BitwiseOR25/1 -> [Byte_25]
  Data Type Conversion65/1 -> BitwiseOR26/1
  [Byte_26_CAN1_ESC_EstVehSpd] -> Data Type Conversion65/1
  BitwiseOR26/1 -> [Byte_26]
  Data Type Conversion66/1 -> BitwiseOR27/1
  [Byte_27_CAN1_ESC_TSA_Active] -> Data Type Conversion66/1
  BitwiseOR27/1 -> [Byte_27]
  constant/1 -> [Byte_28]
  constant1/1 -> [Byte_29]
  constant2/1 -> [Byte_30]
  constant3/1 -> [Byte_31]
  [Byte_1] -> Mux/1
  [Byte_2] -> Mux/2
  [Byte_3] -> Mux/3
  [Byte_4] -> Mux/4
  [Byte_5] -> Mux/5
  [Byte_6] -> Mux/6
  [Byte_7] -> Mux/7
  [Byte_8] -> Mux/8
  [Byte_9] -> Mux/9
  [Byte_10] -> Mux/10
  [Byte_11] -> Mux/11
  [Byte_12] -> Mux/12
  [Byte_13] -> Mux/13
  [Byte_14] -> Mux/14
  [Byte_15] -> Mux/15
  [Byte_16] -> Mux/16
  [Byte_17] -> Mux/17
  [Byte_18] -> Mux/18
  [Byte_19] -> Mux/19
  [Byte_20] -> Mux/20
  [Byte_21] -> Mux/21
  [Byte_22] -> Mux/22
  [Byte_23] -> Mux/23
  [Byte_24] -> Mux/24
  [Byte_25] -> Mux/25
  [Byte_26] -> Mux/26
  [Byte_27] -> Mux/27
  [Byte_28] -> Mux/28
  [Byte_29] -> Mux/29
  [Byte_30] -> Mux/30
  [Byte_31] -> Mux/31
  Mux/1 -> [VHAL_CAN1ESC1noCS_raw]
  KHAL_CAN1ESC1E2E_flg/1 -> DDM_CS&RC_Comparison/1
  0xB3/1 -> DDM_CS&RC_Comparison/2
  0x5F/1 -> DDM_CS&RC_Comparison/3
  [VHAL_CAN1ESC1noCS_raw] -> DDM_CS&RC_Comparison/4
  [Byte_0] -> DDM_CS&RC_Comparison/5
  [RC_ECU] -> DDM_CS&RC_Comparison/6
  MessageRollingCounter/1 -> DDM_CS&RC_Comparison/7
  DDM_CS&RC_Comparison/1 -> VHAL_ESC1CSErr_flg/1
  DDM_CS&RC_Comparison/2 -> VHAL_ESC1RCErr_flg/1
  [DT_CAN1_SG_ESC1] -> bus_selector1/1
  bus_selector1/1 -> ABSActive/1(ABS_Active)  "<CAN1_ABS_Active>"
  ABSActive/1(VHAL_ABSActive_flg) -> VHAL_ABSActive_flg/1
  [DT_CAN1_SG_ESC1] -> bus_selector2/1
  bus_selector2/1 -> ABSFailed/1(ABS_Failed)  "<CAN1_ABS_Failed>"
  ABSFailed/1(VHAL_ABSFailed_flg) -> VHAL_ABSFailed_flg/1
  [DT_CAN1_SG_ESC1] -> bus_selector3/1
  bus_selector3/1 -> ABSWnlmpSta/1(ABS_WnlmpSta)  "<CAN1_ABS_WnlmpSta>"
  ABSWnlmpSta/1(VHAL_ABSWnlmpSta_flg) -> VHAL_ABSWnlmpSta_flg/1
  [DT_CAN1_SG_ESC1] -> bus_selector4/1
  bus_selector4/1 -> AVHActive/1(AVH_Active)  "<CAN1_AVH_Active>"
  AVHActive/1(VHAL_AVHActive_flg) -> VHAL_AVHActive_flg/1
  [DT_CAN1_SG_ESC1] -> bus_selector5/1
  bus_selector5/1 -> AVHFailed/1(AVH_Failed)  "<CAN1_AVH_Failed>"
  AVHFailed/1(VHAL_AVHFailed_flg) -> VHAL_AVHFailed_flg/1
  [DT_CAN1_SG_ESC1] -> bus_selector6/1
  bus_selector6/1 -> AmberWnlmpSta/1(Amber_WnlmpSta)  "<CAN1_Amber_WnlmpSta>"
  AmberWnlmpSta/1(VHAL_AmberWnlmpSta_flg) -> VHAL_AmberWnlmpSta_flg/1
  [DT_CAN1_SG_ESC1] -> bus_selector7/1
  bus_selector7/1 -> BTCSActive/1(BTCS_Active)  "<CAN1_BTCS_Active>"
  BTCSActive/1(VHAL_BTCSActive_flg) -> VHAL_BTCSActive_flg/1
  [DT_CAN1_SG_ESC1] -> bus_selector8/1
  bus_selector8/1 -> EBDActive/1(EBD_Active)  "<CAN1_EBD_Active>"
  EBDActive/1(VHAL_EBDActive_flg) -> VHAL_EBDActive_flg/1
  [DT_CAN1_SG_ESC1] -> bus_selector9/1
  bus_selector9/1 -> EBDFailed/1(EBD_Failed)  "<CAN1_EBD_Failed>"
  EBDFailed/1(VHAL_EBDFailed_flg) -> VHAL_EBDFailed_flg/1
  [DT_CAN1_SG_ESC1] -> bus_selector10/1
  bus_selector10/1 -> ESC1CS/1(ESC1_CS)  "<CAN1_ESC1_CS>"
  ESC1CS/1(VHAL_ESC1CS_enum) -> VHAL_ESC1CS_enum/1
  [DT_CAN1_SG_ESC1] -> bus_selector11/1
  bus_selector11/1 -> ESC1RC/1(ESC1_RC)  "<CAN1_ESC1_RC>"
  ESC1RC/1(VHAL_ESC1RC_enum) -> VHAL_ESC1RC_enum/1, [RC_ECU]
  [DT_CAN1_SG_ESC1] -> bus_selector12/1
  bus_selector12/1 -> ESCActive/1(ESC_Active)  "<CAN1_ESC_Active>"
  ESCActive/1(VHAL_ESCActive_flg) -> VHAL_ESCActive_flg/1
  [DT_CAN1_SG_ESC1] -> bus_selector13/1
  bus_selector13/1 -> ESCBeepReq/1(ESC_BeepReq)  "<CAN1_ESC_BeepReq>"
  ESCBeepReq/1(VHAL_ESCBeepReq_flg) -> VHAL_ESCBeepReq_flg/1
  [DT_CAN1_SG_ESC1] -> bus_selector14/1
  bus_selector14/1 -> ESCFailed/1(ESC_Failed)  "<CAN1_ESC_Failed>"
  ESCFailed/1(VHAL_ESCFailed_flg) -> VHAL_ESCFailed_flg/1
  [DT_CAN1_SG_ESC1] -> bus_selector15/1
  bus_selector15/1 -> ESCOFFStatus/1(ESC_OFF_Status)  "<CAN1_ESC_OFF_Status>"
  ESCOFFStatus/1(VHAL_ESCOFFStatus_enum) -> VHAL_ESCOFFStatus_enum/1
  [DT_CAN1_SG_ESC1] -> bus_selector16/1
  bus_selector16/1 -> ESCOfflmpSta/1(ESC_Off_lmpSta)  "<CAN1_ESC_Off_lmpSta>"
  ESCOfflmpSta/1(VHAL_ESCOfflmpSta_flg) -> VHAL_ESCOfflmpSta_flg/1
  [DT_CAN1_SG_ESC1] -> bus_selector17/1
  bus_selector17/1 -> ESCWnlmpSta/1(ESC_WnlmpSta)  "<CAN1_ESC_WnlmpSta>"
  ESCWnlmpSta/1(VHAL_ESCWnlmpSta_enum) -> VHAL_ESCWnlmpSta_enum/1
  [DT_CAN1_SG_ESC1] -> bus_selector18/1
  bus_selector18/1 -> ESSActive/1(ESS_Active)  "<CAN1_ESS_Active>"
  ESSActive/1(VHAL_ESSActive_flg) -> VHAL_ESSActive_flg/1
  [DT_CAN1_SG_ESC1] -> bus_selector19/1
  bus_selector19/1 -> FrPTCSActive/1(Fr_PTCS_Active)  "<CAN1_Fr_PTCS_Active>"
  FrPTCSActive/1(VHAL_FrPTCSActive_flg) -> VHAL_FrPTCSActive_flg/1
  [DT_CAN1_SG_ESC1] -> bus_selector20/1
  bus_selector20/1 -> FrntAxlTrqReqDrv/1(FrntAxlTrqReq_Drv)  "<CAN1_FrntAxlTrqReq_Drv>"
  FrntAxlTrqReqDrv/1(VHAL_FrntAxlTrqReqDrv_Nm) -> VHAL_FrntAxlTrqReqDrv_Nm/1
  [DT_CAN1_SG_ESC1] -> bus_selector21/1
  bus_selector21/1 -> GRADE/1(GRADE)  "<CAN1_GRADE>"
  GRADE/1(VHAL_GRADE_Deg) -> VHAL_GRADE_Deg/1
  [DT_CAN1_SG_ESC1] -> bus_selector22/1
  bus_selector22/1 -> HBBActive/1(HBB_Active)  "<CAN1_HBB_Active>"
  HBBActive/1(VHAL_HBBActive_flg) -> VHAL_HBBActive_flg/1
  [DT_CAN1_SG_ESC1] -> bus_selector23/1
  bus_selector23/1 -> HBBFailed/1(HBB_Failed)  "<CAN1_HBB_Failed>"
  HBBFailed/1(VHAL_HBBFailed_flg) -> VHAL_HBBFailed_flg/1
  [DT_CAN1_SG_ESC1] -> bus_selector24/1
  bus_selector24/1 -> HDDActive/1(HDD_Active)  "<CAN1_HDD_Active>"
  HDDActive/1(VHAL_HDDActive_flg) -> VHAL_HDDActive_flg/1
  [DT_CAN1_SG_ESC1] -> bus_selector25/1
  bus_selector25/1 -> HDDFailed/1(HDD_Failed)  "<CAN1_HDD_Failed>"
  HDDFailed/1(VHAL_HDDFailed_flg) -> VHAL_HDDFailed_flg/1
  [DT_CAN1_SG_ESC1] -> bus_selector26/1
  bus_selector26/1 -> HSAActive/1(HSA_Active)  "<CAN1_HSA_Active>"
  HSAActive/1(VHAL_HSAActive_flg) -> VHAL_HSAActive_flg/1
  [DT_CAN1_SG_ESC1] -> bus_selector27/1
  bus_selector27/1 -> HSAFailed/1(HSA_Failed)  "<CAN1_HSA_Failed>"
  HSAFailed/1(VHAL_HSAFailed_flg) -> VHAL_HSAFailed_flg/1
  [DT_CAN1_SG_ESC1] -> bus_selector28/1
  bus_selector28/1 -> LFPulseCount/1(LF_PulseCount)  "<CAN1_LF_PulseCount>"
  LFPulseCount/1(VHAL_LFPulseCount_enum) -> VHAL_LFPulseCount_enum/1
  [DT_CAN1_SG_ESC1] -> bus_selector29/1
  bus_selector29/1 -> LFPulseCountV/1(LF_PulseCount_V)  "<CAN1_LF_PulseCount_V>"
  LFPulseCountV/1(VHAL_LFPulseCountV_flg) -> VHAL_LFPulseCountV_flg/1
  [DT_CAN1_SG_ESC1] -> bus_selector30/1
  bus_selector30/1 -> LFRawWhlSpeed/1(LF_RawWhlSpeed)  "<CAN1_LF_RawWhlSpeed>"
  LFRawWhlSpeed/1(VHAL_LFRawWhlSpeed_kph) -> VHAL_LFRawWhlSpeed_kph/1
  [DT_CAN1_SG_ESC1] -> bus_selector31/1
  bus_selector31/1 -> LFRawWhlSpeedV/1(LF_RawWhlSpeed_V)  "<CAN1_LF_RawWhlSpeed_V>"
  LFRawWhlSpeedV/1(VHAL_LFRawWhlSpeedV_flg) -> VHAL_LFRawWhlSpeedV_flg/1
  [DT_CAN1_SG_ESC1] -> bus_selector32/1
  bus_selector32/1 -> LFWhlRotDir/1(LF_WhlRotDir)  "<CAN1_LF_WhlRotDir>"
  LFWhlRotDir/1(VHAL_LFWhlRotDir_enum) -> VHAL_LFWhlRotDir_enum/1
  [DT_CAN1_SG_ESC1] -> bus_selector33/1
  bus_selector33/1 -> LRPulseCount/1(LR_PulseCount)  "<CAN1_LR_PulseCount>"
  LRPulseCount/1(VHAL_LRPulseCount_enum) -> VHAL_LRPulseCount_enum/1
  [DT_CAN1_SG_ESC1] -> bus_selector34/1
  bus_selector34/1 -> LRPulseCountV/1(LR_PulseCount_V)  "<CAN1_LR_PulseCount_V>"
  LRPulseCountV/1(VHAL_LRPulseCountV_flg) -> VHAL_LRPulseCountV_flg/1
  [DT_CAN1_SG_ESC1] -> bus_selector35/1
  bus_selector35/1 -> LRRawWhlSpeed/1(LR_RawWhlSpeed)  "<CAN1_LR_RawWhlSpeed>"
  LRRawWhlSpeed/1(VHAL_LRRawWhlSpeed_kph) -> VHAL_LRRawWhlSpeed_kph/1
  [DT_CAN1_SG_ESC1] -> bus_selector36/1
  bus_selector36/1 -> LRRawWhlSpeedV/1(LR_RawWhlSpeed_V)  "<CAN1_LR_RawWhlSpeed_V>"
  LRRawWhlSpeedV/1(VHAL_LRRawWhlSpeedV_flg) -> VHAL_LRRawWhlSpeedV_flg/1
  [DT_CAN1_SG_ESC1] -> bus_selector37/1
  bus_selector37/1 -> LRWhlRotDir/1(LR_WhlRotDir)  "<CAN1_LR_WhlRotDir>"
  LRWhlRotDir/1(VHAL_LRWhlRotDir_enum) -> VHAL_LRWhlRotDir_enum/1
  [DT_CAN1_SG_ESC1] -> bus_selector38/1
  bus_selector38/1 -> PBAActive/1(PBA_Active)  "<CAN1_PBA_Active>"
  PBAActive/1(VHAL_PBAActive_flg) -> VHAL_PBAActive_flg/1
  [DT_CAN1_SG_ESC1] -> bus_selector39/1
  bus_selector39/1 -> PBAFailed/1(PBA_Failed)  "<CAN1_PBA_Failed>"
  PBAFailed/1(VHAL_PBAFailed_flg) -> VHAL_PBAFailed_flg/1
  [DT_CAN1_SG_ESC1] -> bus_selector40/1
  bus_selector40/1 -> RFPulseCount/1(RF_PulseCount)  "<CAN1_RF_PulseCount>"
  RFPulseCount/1(VHAL_RFPulseCount_enum) -> VHAL_RFPulseCount_enum/1
  [DT_CAN1_SG_ESC1] -> bus_selector41/1
  bus_selector41/1 -> RFPulseCountV/1(RF_PulseCount_V)  "<CAN1_RF_PulseCount_V>"
  RFPulseCountV/1(VHAL_RFPulseCountV_flg) -> VHAL_RFPulseCountV_flg/1
  [DT_CAN1_SG_ESC1] -> bus_selector42/1
  bus_selector42/1 -> RFRawWhlSpeed/1(RF_RawWhlSpeed)  "<CAN1_RF_RawWhlSpeed>"
  RFRawWhlSpeed/1(VHAL_RFRawWhlSpeed_kph) -> VHAL_RFRawWhlSpeed_kph/1
  [DT_CAN1_SG_ESC1] -> bus_selector43/1
  bus_selector43/1 -> RFRawWhlSpeedV/1(RF_RawWhlSpeed_V)  "<CAN1_RF_RawWhlSpeed_V>"
  RFRawWhlSpeedV/1(VHAL_RFRawWhlSpeedV_flg) -> VHAL_RFRawWhlSpeedV_flg/1
  [DT_CAN1_SG_ESC1] -> bus_selector44/1
  bus_selector44/1 -> RFWhlRotDir/1(RF_WhlRotDir)  "<CAN1_RF_WhlRotDir>"
  RFWhlRotDir/1(VHAL_RFWhlRotDir_enum) -> VHAL_RFWhlRotDir_enum/1
  [DT_CAN1_SG_ESC1] -> bus_selector45/1
  bus_selector45/1 -> RRPulseCount/1(RR_PulseCount)  "<CAN1_RR_PulseCount>"
  RRPulseCount/1(VHAL_RRPulseCount_enum) -> VHAL_RRPulseCount_enum/1
  [DT_CAN1_SG_ESC1] -> bus_selector46/1
  bus_selector46/1 -> RRPulseCountV/1(RR_PulseCount_V)  "<CAN1_RR_PulseCount_V>"
  RRPulseCountV/1(VHAL_RRPulseCountV_flg) -> VHAL_RRPulseCountV_flg/1
  [DT_CAN1_SG_ESC1] -> bus_selector47/1
  bus_selector47/1 -> RRRawWhlSpeed/1(RR_RawWhlSpeed)  "<CAN1_RR_RawWhlSpeed>"
  RRRawWhlSpeed/1(VHAL_RRRawWhlSpeed_kph) -> VHAL_RRRawWhlSpeed_kph/1
  [DT_CAN1_SG_ESC1] -> bus_selector48/1
  bus_selector48/1 -> RRRawWhlSpeedV/1(RR_RawWhlSpeed_V)  "<CAN1_RR_RawWhlSpeed_V>"
  RRRawWhlSpeedV/1(VHAL_RRRawWhlSpeedV_flg) -> VHAL_RRRawWhlSpeedV_flg/1
  [DT_CAN1_SG_ESC1] -> bus_selector49/1
  bus_selector49/1 -> RRWhlRotDir/1(RR_WhlRotDir)  "<CAN1_RR_WhlRotDir>"
  RRWhlRotDir/1(VHAL_RRWhlRotDir_enum) -> VHAL_RRWhlRotDir_enum/1
  [DT_CAN1_SG_ESC1] -> bus_selector50/1
  bus_selector50/1 -> RearAxlTrqReqDrv/1(RearAxlTrqReq_Drv)  "<CAN1_RearAxlTrqReq_Drv>"
  RearAxlTrqReqDrv/1(VHAL_RearAxlTrqReqDrv_Nm) -> VHAL_RearAxlTrqReqDrv_Nm/1
  [DT_CAN1_SG_ESC1] -> bus_selector51/1
  bus_selector51/1 -> RedWnlmpSta/1(Red_WnlmpSta)  "<CAN1_Red_WnlmpSta>"
  RedWnlmpSta/1(VHAL_RedWnlmpSta_flg) -> VHAL_RedWnlmpSta_flg/1
  [DT_CAN1_SG_ESC1] -> bus_selector52/1
  bus_selector52/1 -> RrPTCSActive/1(Rr_PTCS_Active)  "<CAN1_Rr_PTCS_Active>"
  RrPTCSActive/1(VHAL_RrPTCSActive_flg) -> VHAL_RrPTCSActive_flg/1
  [DT_CAN1_SG_ESC1] -> bus_selector53/1
  bus_selector53/1 -> TCSActive/1(TCS_Active)  "<CAN1_TCS_Active>"
  TCSActive/1(VHAL_TCSActive_flg) -> VHAL_TCSActive_flg/1
  [DT_CAN1_SG_ESC1] -> bus_selector54/1
  bus_selector54/1 -> TCSFailed/1(TCS_Failed)  "<CAN1_TCS_Failed>"
  TCSFailed/1(VHAL_TCSFailed_flg) -> VHAL_TCSFailed_flg/1
  [DT_CAN1_SG_ESC1] -> bus_selector55/1
  bus_selector55/1 -> VehSpeed/1(VehSpeed)  "<CAN1_VehSpeed>"
  VehSpeed/1(VHAL_VehSpeed_kph) -> VHAL_VehSpeed_kph/1
